simulink model "Dyn3DoF_astro"  (R2018b)
settings: configuration reference "Configuration" (kept outside this file)
model workspace (MATLAB code in the model file):
  | CON = Simulink.Parameter;
  | CON.DataType = 'Bus: Bus_CON';
  | CON.Value = Simulink.Bus.createMATLABStruct('Bus_CON');
settings Model: ParameterArgumentNames=CON  OrderedModelArguments=off  Creator=Ethan  LastModifiedBy=Ethan
settings ConfigSetRef: SourceLocation=Base Workspace

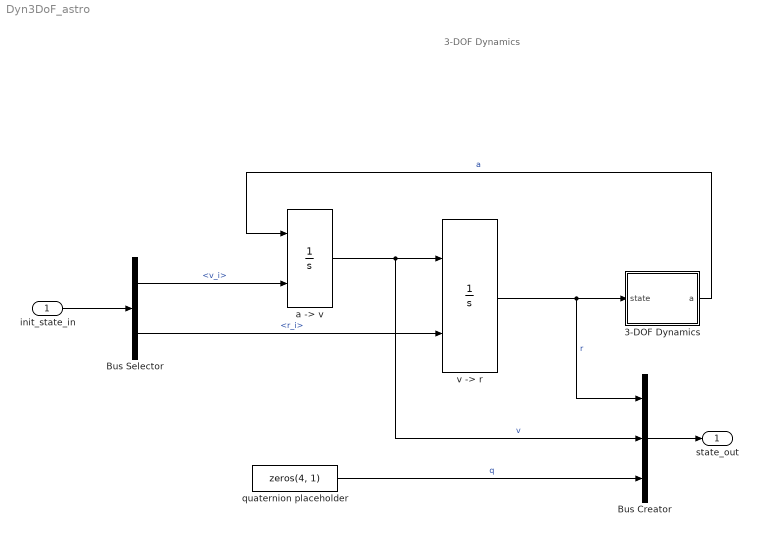
== system Dyn3DoF_astro ==
  note: 3-DOF Dynamics
  init_state_in : Inport  OutDataTypeStr=Bus: Bus_state
  3-DOF Dynamics : MATLAB Function  TreatAsAtomicUnit=on
  Bus Creator : BusCreator  Inputs=3  OutDataTypeStr=Bus: Bus_state  NonVirtualBus=on
      settings: InheritFromInputs=off
  Bus Selector : BusSelector  OutputSignals=v_i,r_i
  "a -> v" : Integrator  InitialConditionSource=external
  quaternion placeholder : Constant  Value=zeros(4, 1)
  "v -> r" : Integrator  InitialConditionSource=external
  state_out : Outport  OutDataTypeStr=Bus: Bus_state
  wires:
  init_state_in/1 -> Bus Selector/1
  "v -> r"/1 -> Bus Creator/1, 3-DOF Dynamics/1(state)  "r"
  Bus Selector/1 -> "a -> v"/2  "<v_i>"
  Bus Selector/2 -> "v -> r"/2  "<r_i>"
  3-DOF Dynamics/1(a) -> "a -> v"/1  "a"
  "a -> v"/1 -> Bus Creator/2, "v -> r"/1  "v"
  quaternion placeholder/1 -> Bus Creator/3  "q"
  Bus Creator/1 -> state_out/1

== matlab function Dyn3DoF_astro/3-DOF Dynamics ==
  data: state input; a output; CON parameter
function a = dyn(state, CON)

r = state(1:3);

a = - CON.mu * r / norm(r) ^ 3;

end
